simulink model "Timers"  (R2025a)
settings: Solver=FixedStepDiscrete  StartTime=0  StopTime=1  FixedStep=1e-7  RelTol=1e-3
libraries: simulink_extras x216, simulink x13
(part 4 of 7)

== system Timers/Eg: Prescaler/Counter ==
  INC : Inport
  TC_RST : Inport  Port=2
  Constant : Constant
  D Flip-Flop{1..7,11} (8 alike) : simulink_extras/Flip Flops/D Flip-Flop
  Delay One Step : Delay  DelayLength=1
  Demux : Demux  Outputs=8
  Half Adder : Subsystem
      settings: PortSchema="{\"entries\":[{\"content\":{\"sides\":[{\"content\":{\"connectorIds\":[\"In1\"]},\"type\":\"ConnectorPlacement.EquallySpacedRectSide\",\"uuid\":\"d3a7e232-15f2-47a9-a065-9480c81dc57e\"},{\"content\":{\"connectorIds\":[\"Out1\"],\"side\":\"RIGHT\"},\"type\":\"ConnectorPlacement.EquallySpacedRectSide\",\"uuid\":\"e118f150-fee7-4aeb-941e-53c3f02c6791\"},{\"content\":{\"connectorIds\":[\"Out2\"],\"side\":\"TOP\"},\"type\":\"ConnectorPlacement.EquallySpacedRectSide\",\"uuid\":\"6d9038ab-faad-455b-a9c5-8fe0bbf34e51\"},{\"content\":{\"connectorIds\":[\"In2\"],\"side\":\"BOTTOM\"},\"type\":\"ConnectorPlacement.EquallySpacedRectSide\",\"uuid\":\"d09c8d4f-08f3-4c52-88a6-8c6db517fc7a\"}]},\"type\":\"ConnectorPlacement.EquallySpacedConnector\",\"uuid\":\"5bc947ce-f1cd-4957-9186-40c14c78de7d\"}],\"packageUris\":[\"http://schema.mathworks.com/mf0/Connector/R2020b\"],\"version\":\"1.0\"}"
  Half Adder1 : Subsystem
      settings: PortSchema="{\"entries\":[{\"content\":{\"sides\":[{\"content\":{\"connectorIds\":[\"In1\"]},\"type\":\"ConnectorPlacement.EquallySpacedRectSide\",\"uuid\":\"d3a7e232-15f2-47a9-a065-9480c81dc57e\"},{\"content\":{\"connectorIds\":[\"Out1\"],\"side\":\"RIGHT\"},\"type\":\"ConnectorPlacement.EquallySpacedRectSide\",\"uuid\":\"e118f150-fee7-4aeb-941e-53c3f02c6791\"},{\"content\":{\"connectorIds\":[\"Out2\"],\"side\":\"TOP\"},\"type\":\"ConnectorPlacement.EquallySpacedRectSide\",\"uuid\":\"6d9038ab-faad-455b-a9c5-8fe0bbf34e51\"},{\"content\":{\"connectorIds\":[\"In2\"],\"side\":\"BOTTOM\"},\"type\":\"ConnectorPlacement.EquallySpacedRectSide\",\"uuid\":\"d09c8d4f-08f3-4c52-88a6-8c6db517fc7a\"}]},\"type\":\"ConnectorPlacement.EquallySpacedConnector\",\"uuid\":\"5bc947ce-f1cd-4957-9186-40c14c78de7d\"}],\"packageUris\":[\"http://schema.mathworks.com/mf0/Connector/R2020b\"],\"version\":\"1.0\"}"
  Half Adder2 : Subsystem
      settings: PortSchema="{\"entries\":[{\"content\":{\"sides\":[{\"content\":{\"connectorIds\":[\"In1\"]},\"type\":\"ConnectorPlacement.EquallySpacedRectSide\",\"uuid\":\"d3a7e232-15f2-47a9-a065-9480c81dc57e\"},{\"content\":{\"connectorIds\":[\"Out1\"],\"side\":\"RIGHT\"},\"type\":\"ConnectorPlacement.EquallySpacedRectSide\",\"uuid\":\"e118f150-fee7-4aeb-941e-53c3f02c6791\"},{\"content\":{\"connectorIds\":[\"Out2\"],\"side\":\"TOP\"},\"type\":\"ConnectorPlacement.EquallySpacedRectSide\",\"uuid\":\"6d9038ab-faad-455b-a9c5-8fe0bbf34e51\"},{\"content\":{\"connectorIds\":[\"In2\"],\"side\":\"BOTTOM\"},\"type\":\"ConnectorPlacement.EquallySpacedRectSide\",\"uuid\":\"d09c8d4f-08f3-4c52-88a6-8c6db517fc7a\"}]},\"type\":\"ConnectorPlacement.EquallySpacedConnector\",\"uuid\":\"5bc947ce-f1cd-4957-9186-40c14c78de7d\"}],\"packageUris\":[\"http://schema.mathworks.com/mf0/Connector/R2020b\"],\"version\":\"1.0\"}"
  Half Adder3 : Subsystem
      settings: PortSchema="{\"entries\":[{\"content\":{\"sides\":[{\"content\":{\"connectorIds\":[\"In1\"]},\"type\":\"ConnectorPlacement.EquallySpacedRectSide\",\"uuid\":\"d3a7e232-15f2-47a9-a065-9480c81dc57e\"},{\"content\":{\"connectorIds\":[\"Out1\"],\"side\":\"RIGHT\"},\"type\":\"ConnectorPlacement.EquallySpacedRectSide\",\"uuid\":\"e118f150-fee7-4aeb-941e-53c3f02c6791\"},{\"content\":{\"connectorIds\":[\"Out2\"],\"side\":\"TOP\"},\"type\":\"ConnectorPlacement.EquallySpacedRectSide\",\"uuid\":\"6d9038ab-faad-455b-a9c5-8fe0bbf34e51\"},{\"content\":{\"connectorIds\":[\"In2\"],\"side\":\"BOTTOM\"},\"type\":\"ConnectorPlacement.EquallySpacedRectSide\",\"uuid\":\"d09c8d4f-08f3-4c52-88a6-8c6db517fc7a\"}]},\"type\":\"ConnectorPlacement.EquallySpacedConnector\",\"uuid\":\"5bc947ce-f1cd-4957-9186-40c14c78de7d\"}],\"packageUris\":[\"http://schema.mathworks.com/mf0/Connector/R2020b\"],\"version\":\"1.0\"}"
  Half Adder4 : Subsystem
      settings: PortSchema="{\"entries\":[{\"content\":{\"sides\":[{\"content\":{\"connectorIds\":[\"In1\"]},\"type\":\"ConnectorPlacement.EquallySpacedRectSide\",\"uuid\":\"d3a7e232-15f2-47a9-a065-9480c81dc57e\"},{\"content\":{\"connectorIds\":[\"Out1\"],\"side\":\"RIGHT\"},\"type\":\"ConnectorPlacement.EquallySpacedRectSide\",\"uuid\":\"e118f150-fee7-4aeb-941e-53c3f02c6791\"},{\"content\":{\"connectorIds\":[\"Out2\"],\"side\":\"TOP\"},\"type\":\"ConnectorPlacement.EquallySpacedRectSide\",\"uuid\":\"6d9038ab-faad-455b-a9c5-8fe0bbf34e51\"},{\"content\":{\"connectorIds\":[\"In2\"],\"side\":\"BOTTOM\"},\"type\":\"ConnectorPlacement.EquallySpacedRectSide\",\"uuid\":\"d09c8d4f-08f3-4c52-88a6-8c6db517fc7a\"}]},\"type\":\"ConnectorPlacement.EquallySpacedConnector\",\"uuid\":\"5bc947ce-f1cd-4957-9186-40c14c78de7d\"}],\"packageUris\":[\"http://schema.mathworks.com/mf0/Connector/R2020b\"],\"version\":\"1.0\"}"
  Half Adder5 : Subsystem
      settings: PortSchema="{\"entries\":[{\"content\":{\"sides\":[{\"content\":{\"connectorIds\":[\"In1\"]},\"type\":\"ConnectorPlacement.EquallySpacedRectSide\",\"uuid\":\"d3a7e232-15f2-47a9-a065-9480c81dc57e\"},{\"content\":{\"connectorIds\":[\"Out1\"],\"side\":\"RIGHT\"},\"type\":\"ConnectorPlacement.EquallySpacedRectSide\",\"uuid\":\"e118f150-fee7-4aeb-941e-53c3f02c6791\"},{\"content\":{\"connectorIds\":[\"Out2\"],\"side\":\"TOP\"},\"type\":\"ConnectorPlacement.EquallySpacedRectSide\",\"uuid\":\"6d9038ab-faad-455b-a9c5-8fe0bbf34e51\"},{\"content\":{\"connectorIds\":[\"In2\"],\"side\":\"BOTTOM\"},\"type\":\"ConnectorPlacement.EquallySpacedRectSide\",\"uuid\":\"d09c8d4f-08f3-4c52-88a6-8c6db517fc7a\"}]},\"type\":\"ConnectorPlacement.EquallySpacedConnector\",\"uuid\":\"5bc947ce-f1cd-4957-9186-40c14c78de7d\"}],\"packageUris\":[\"http://schema.mathworks.com/mf0/Connector/R2020b\"],\"version\":\"1.0\"}"
  Half Adder6 : Subsystem
      settings: PortSchema="{\"entries\":[{\"content\":{\"sides\":[{\"content\":{\"connectorIds\":[\"In1\"]},\"type\":\"ConnectorPlacement.EquallySpacedRectSide\",\"uuid\":\"d3a7e232-15f2-47a9-a065-9480c81dc57e\"},{\"content\":{\"connectorIds\":[\"Out1\"],\"side\":\"RIGHT\"},\"type\":\"ConnectorPlacement.EquallySpacedRectSide\",\"uuid\":\"e118f150-fee7-4aeb-941e-53c3f02c6791\"},{\"content\":{\"side\":\"TOP\"},\"type\":\"ConnectorPlacement.EquallySpacedRectSide\",\"uuid\":\"6d9038ab-faad-455b-a9c5-8fe0bbf34e51\"},{\"content\":{\"connectorIds\":[\"In2\"],\"side\":\"BOTTOM\"},\"type\":\"ConnectorPlacement.EquallySpacedRectSide\",\"uuid\":\"d09c8d4f-08f3-4c52-88a6-8c6db517fc7a\"}]},\"type\":\"ConnectorPlacement.EquallySpacedConnector\",\"uuid\":\"5bc947ce-f1cd-4957-9186-40c14c78de7d\"}],\"packageUris\":[\"http://schema.mathworks.com/mf0/Connector/R2020b\"],\"version\":\"1.0\"}"
  Half Adder7 : Subsystem
      settings: PortSchema="{\"entries\":[{\"content\":{\"sides\":[{\"content\":{\"connectorIds\":[\"In1\"]},\"type\":\"ConnectorPlacement.EquallySpacedRectSide\",\"uuid\":\"d3a7e232-15f2-47a9-a065-9480c81dc57e\"},{\"content\":{\"connectorIds\":[\"Out1\"],\"side\":\"RIGHT\"},\"type\":\"ConnectorPlacement.EquallySpacedRectSide\",\"uuid\":\"e118f150-fee7-4aeb-941e-53c3f02c6791\"},{\"content\":{\"connectorIds\":[\"Out2\"],\"side\":\"TOP\"},\"type\":\"ConnectorPlacement.EquallySpacedRectSide\",\"uuid\":\"6d9038ab-faad-455b-a9c5-8fe0bbf34e51\"},{\"content\":{\"connectorIds\":[\"In2\"],\"side\":\"BOTTOM\"},\"type\":\"ConnectorPlacement.EquallySpacedRectSide\",\"uuid\":\"d09c8d4f-08f3-4c52-88a6-8c6db517fc7a\"}]},\"type\":\"ConnectorPlacement.EquallySpacedConnector\",\"uuid\":\"5bc947ce-f1cd-4957-9186-40c14c78de7d\"}],\"packageUris\":[\"http://schema.mathworks.com/mf0/Connector/R2020b\"],\"version\":\"1.0\"}"
  Mux1 : Mux  Inputs=8
  Mux2 : Mux  Inputs=8
  NOT : Logic  Operator=NOT  IconShape=distinctive  AllPortsSameDT=off  OutDataTypeStr=boolean
  TC : Outport
  wires:
  Mux1/1 -> Delay One Step/1
  TC_RST/1 -> NOT/1
  Delay One Step/1 -> Demux/1
  Demux/4 -> D Flip-Flop4/1
  Demux/3 -> D Flip-Flop2/1
  Demux/2 -> D Flip-Flop3/1
  Demux/1 -> D Flip-Flop1/1
  Demux/8 -> D Flip-Flop7/1
  Demux/7 -> D Flip-Flop5/1
  Demux/6 -> D Flip-Flop6/1
  Demux/5 -> D Flip-Flop11/1
  INC/1 -> D Flip-Flop2/2, D Flip-Flop3/2, D Flip-Flop1/2, D Flip-Flop4/2, D Flip-Flop11/2, D Flip-Flop6/2, D Flip-Flop5/2, D Flip-Flop7/2
  Constant/1 -> Half Adder7/2("B ")
  Half Adder5/2(Carry) -> Half Adder6/2("B ")
  Half Adder/2(Carry) -> Half Adder1/2("B ")
  Half Adder4/1(Sum) -> Mux1/3
  Half Adder6/1(Sum) -> Mux1/1
  Half Adder5/1(Sum) -> Mux1/2
  Half Adder1/1(Sum) -> Mux1/6
  Half Adder/1(Sum) -> Mux1/7
  Half Adder2/1(Sum) -> Mux1/5
  Half Adder2/2(Carry) -> Half Adder3/2("B ")
  Half Adder3/1(Sum) -> Mux1/4
  Half Adder4/2(Carry) -> Half Adder5/2("B ")
  Half Adder3/2(Carry) -> Half Adder4/2("B ")
  Half Adder1/2(Carry) -> Half Adder2/2("B ")
  Half Adder7/1(Sum) -> Mux1/8
  Half Adder7/2(Carry) -> Half Adder/2("B ")
  D Flip-Flop1/1 -> Mux2/1, Half Adder6/1(A)  "D1"
  D Flip-Flop3/1 -> Mux2/2, Half Adder5/1(A)  "D3"
  D Flip-Flop2/1 -> Mux2/3, Half Adder4/1(A)  "D4"
  D Flip-Flop4/1 -> Mux2/4, Half Adder3/1(A)  "D2"
  D Flip-Flop11/1 -> Mux2/5, Half Adder2/1(A)  "D1"
  D Flip-Flop6/1 -> Mux2/6, Half Adder1/1(A)  "D3"
  D Flip-Flop5/1 -> Mux2/7, Half Adder/1(A)  "D4"
  D Flip-Flop7/1 -> Mux2/8, Half Adder7/1(A)  "D2"
  Mux2/1 -> TC/1
  NOT/1 -> D Flip-Flop2/3, D Flip-Flop1/3, D Flip-Flop3/3, D Flip-Flop4/3, D Flip-Flop11/3, D Flip-Flop6/3, D Flip-Flop5/3, D Flip-Flop7/3

== system Timers/Eg: Prescaler/Counter1 ==
  INC : Inport
  TC_RST : Inport  Port=2
  Constant : Constant
  D Flip-Flop{1..7,11} (8 alike) : simulink_extras/Flip Flops/D Flip-Flop
  Demux : Demux  Outputs=8
  Half Adder : Subsystem
      settings: PortSchema="{\"entries\":[{\"content\":{\"sides\":[{\"content\":{\"connectorIds\":[\"In1\"]},\"type\":\"ConnectorPlacement.EquallySpacedRectSide\",\"uuid\":\"d3a7e232-15f2-47a9-a065-9480c81dc57e\"},{\"content\":{\"connectorIds\":[\"Out1\"],\"side\":\"RIGHT\"},\"type\":\"ConnectorPlacement.EquallySpacedRectSide\",\"uuid\":\"e118f150-fee7-4aeb-941e-53c3f02c6791\"},{\"content\":{\"connectorIds\":[\"Out2\"],\"side\":\"TOP\"},\"type\":\"ConnectorPlacement.EquallySpacedRectSide\",\"uuid\":\"6d9038ab-faad-455b-a9c5-8fe0bbf34e51\"},{\"content\":{\"connectorIds\":[\"In2\"],\"side\":\"BOTTOM\"},\"type\":\"ConnectorPlacement.EquallySpacedRectSide\",\"uuid\":\"d09c8d4f-08f3-4c52-88a6-8c6db517fc7a\"}]},\"type\":\"ConnectorPlacement.EquallySpacedConnector\",\"uuid\":\"5bc947ce-f1cd-4957-9186-40c14c78de7d\"}],\"packageUris\":[\"http://schema.mathworks.com/mf0/Connector/R2020b\"],\"version\":\"1.0\"}"
  Half Adder1 : Subsystem
      settings: PortSchema="{\"entries\":[{\"content\":{\"sides\":[{\"content\":{\"connectorIds\":[\"In1\"]},\"type\":\"ConnectorPlacement.EquallySpacedRectSide\",\"uuid\":\"d3a7e232-15f2-47a9-a065-9480c81dc57e\"},{\"content\":{\"connectorIds\":[\"Out1\"],\"side\":\"RIGHT\"},\"type\":\"ConnectorPlacement.EquallySpacedRectSide\",\"uuid\":\"e118f150-fee7-4aeb-941e-53c3f02c6791\"},{\"content\":{\"connectorIds\":[\"Out2\"],\"side\":\"TOP\"},\"type\":\"ConnectorPlacement.EquallySpacedRectSide\",\"uuid\":\"6d9038ab-faad-455b-a9c5-8fe0bbf34e51\"},{\"content\":{\"connectorIds\":[\"In2\"],\"side\":\"BOTTOM\"},\"type\":\"ConnectorPlacement.EquallySpacedRectSide\",\"uuid\":\"d09c8d4f-08f3-4c52-88a6-8c6db517fc7a\"}]},\"type\":\"ConnectorPlacement.EquallySpacedConnector\",\"uuid\":\"5bc947ce-f1cd-4957-9186-40c14c78de7d\"}],\"packageUris\":[\"http://schema.mathworks.com/mf0/Connector/R2020b\"],\"version\":\"1.0\"}"
  Half Adder2 : Subsystem
      settings: PortSchema="{\"entries\":[{\"content\":{\"sides\":[{\"content\":{\"connectorIds\":[\"In1\"]},\"type\":\"ConnectorPlacement.EquallySpacedRectSide\",\"uuid\":\"d3a7e232-15f2-47a9-a065-9480c81dc57e\"},{\"content\":{\"connectorIds\":[\"Out1\"],\"side\":\"RIGHT\"},\"type\":\"ConnectorPlacement.EquallySpacedRectSide\",\"uuid\":\"e118f150-fee7-4aeb-941e-53c3f02c6791\"},{\"content\":{\"connectorIds\":[\"Out2\"],\"side\":\"TOP\"},\"type\":\"ConnectorPlacement.EquallySpacedRectSide\",\"uuid\":\"6d9038ab-faad-455b-a9c5-8fe0bbf34e51\"},{\"content\":{\"connectorIds\":[\"In2\"],\"side\":\"BOTTOM\"},\"type\":\"ConnectorPlacement.EquallySpacedRectSide\",\"uuid\":\"d09c8d4f-08f3-4c52-88a6-8c6db517fc7a\"}]},\"type\":\"ConnectorPlacement.EquallySpacedConnector\",\"uuid\":\"5bc947ce-f1cd-4957-9186-40c14c78de7d\"}],\"packageUris\":[\"http://schema.mathworks.com/mf0/Connector/R2020b\"],\"version\":\"1.0\"}"
  Half Adder3 : Subsystem
      settings: PortSchema="{\"entries\":[{\"content\":{\"sides\":[{\"content\":{\"connectorIds\":[\"In1\"]},\"type\":\"ConnectorPlacement.EquallySpacedRectSide\",\"uuid\":\"d3a7e232-15f2-47a9-a065-9480c81dc57e\"},{\"content\":{\"connectorIds\":[\"Out1\"],\"side\":\"RIGHT\"},\"type\":\"ConnectorPlacement.EquallySpacedRectSide\",\"uuid\":\"e118f150-fee7-4aeb-941e-53c3f02c6791\"},{\"content\":{\"connectorIds\":[\"Out2\"],\"side\":\"TOP\"},\"type\":\"ConnectorPlacement.EquallySpacedRectSide\",\"uuid\":\"6d9038ab-faad-455b-a9c5-8fe0bbf34e51\"},{\"content\":{\"connectorIds\":[\"In2\"],\"side\":\"BOTTOM\"},\"type\":\"ConnectorPlacement.EquallySpacedRectSide\",\"uuid\":\"d09c8d4f-08f3-4c52-88a6-8c6db517fc7a\"}]},\"type\":\"ConnectorPlacement.EquallySpacedConnector\",\"uuid\":\"5bc947ce-f1cd-4957-9186-40c14c78de7d\"}],\"packageUris\":[\"http://schema.mathworks.com/mf0/Connector/R2020b\"],\"version\":\"1.0\"}"
  Half Adder4 : Subsystem
      settings: PortSchema="{\"entries\":[{\"content\":{\"sides\":[{\"content\":{\"connectorIds\":[\"In1\"]},\"type\":\"ConnectorPlacement.EquallySpacedRectSide\",\"uuid\":\"d3a7e232-15f2-47a9-a065-9480c81dc57e\"},{\"content\":{\"connectorIds\":[\"Out1\"],\"side\":\"RIGHT\"},\"type\":\"ConnectorPlacement.EquallySpacedRectSide\",\"uuid\":\"e118f150-fee7-4aeb-941e-53c3f02c6791\"},{\"content\":{\"connectorIds\":[\"Out2\"],\"side\":\"TOP\"},\"type\":\"ConnectorPlacement.EquallySpacedRectSide\",\"uuid\":\"6d9038ab-faad-455b-a9c5-8fe0bbf34e51\"},{\"content\":{\"connectorIds\":[\"In2\"],\"side\":\"BOTTOM\"},\"type\":\"ConnectorPlacement.EquallySpacedRectSide\",\"uuid\":\"d09c8d4f-08f3-4c52-88a6-8c6db517fc7a\"}]},\"type\":\"ConnectorPlacement.EquallySpacedConnector\",\"uuid\":\"5bc947ce-f1cd-4957-9186-40c14c78de7d\"}],\"packageUris\":[\"http://schema.mathworks.com/mf0/Connector/R2020b\"],\"version\":\"1.0\"}"
  Half Adder5 : Subsystem
      settings: PortSchema="{\"entries\":[{\"content\":{\"sides\":[{\"content\":{\"connectorIds\":[\"In1\"]},\"type\":\"ConnectorPlacement.EquallySpacedRectSide\",\"uuid\":\"d3a7e232-15f2-47a9-a065-9480c81dc57e\"},{\"content\":{\"connectorIds\":[\"Out1\"],\"side\":\"RIGHT\"},\"type\":\"ConnectorPlacement.EquallySpacedRectSide\",\"uuid\":\"e118f150-fee7-4aeb-941e-53c3f02c6791\"},{\"content\":{\"connectorIds\":[\"Out2\"],\"side\":\"TOP\"},\"type\":\"ConnectorPlacement.EquallySpacedRectSide\",\"uuid\":\"6d9038ab-faad-455b-a9c5-8fe0bbf34e51\"},{\"content\":{\"connectorIds\":[\"In2\"],\"side\":\"BOTTOM\"},\"type\":\"ConnectorPlacement.EquallySpacedRectSide\",\"uuid\":\"d09c8d4f-08f3-4c52-88a6-8c6db517fc7a\"}]},\"type\":\"ConnectorPlacement.EquallySpacedConnector\",\"uuid\":\"5bc947ce-f1cd-4957-9186-40c14c78de7d\"}],\"packageUris\":[\"http://schema.mathworks.com/mf0/Connector/R2020b\"],\"version\":\"1.0\"}"
  Half Adder6 : Subsystem
      settings: PortSchema="{\"entries\":[{\"content\":{\"sides\":[{\"content\":{\"connectorIds\":[\"In1\"]},\"type\":\"ConnectorPlacement.EquallySpacedRectSide\",\"uuid\":\"d3a7e232-15f2-47a9-a065-9480c81dc57e\"},{\"content\":{\"connectorIds\":[\"Out1\"],\"side\":\"RIGHT\"},\"type\":\"ConnectorPlacement.EquallySpacedRectSide\",\"uuid\":\"e118f150-fee7-4aeb-941e-53c3f02c6791\"},{\"content\":{\"side\":\"TOP\"},\"type\":\"ConnectorPlacement.EquallySpacedRectSide\",\"uuid\":\"6d9038ab-faad-455b-a9c5-8fe0bbf34e51\"},{\"content\":{\"connectorIds\":[\"In2\"],\"side\":\"BOTTOM\"},\"type\":\"ConnectorPlacement.EquallySpacedRectSide\",\"uuid\":\"d09c8d4f-08f3-4c52-88a6-8c6db517fc7a\"}]},\"type\":\"ConnectorPlacement.EquallySpacedConnector\",\"uuid\":\"5bc947ce-f1cd-4957-9186-40c14c78de7d\"}],\"packageUris\":[\"http://schema.mathworks.com/mf0/Connector/R2020b\"],\"version\":\"1.0\"}"
  Half Adder7 : Subsystem
      settings: PortSchema="{\"entries\":[{\"content\":{\"sides\":[{\"content\":{\"connectorIds\":[\"In1\"]},\"type\":\"ConnectorPlacement.EquallySpacedRectSide\",\"uuid\":\"d3a7e232-15f2-47a9-a065-9480c81dc57e\"},{\"content\":{\"connectorIds\":[\"Out1\"],\"side\":\"RIGHT\"},\"type\":\"ConnectorPlacement.EquallySpacedRectSide\",\"uuid\":\"e118f150-fee7-4aeb-941e-53c3f02c6791\"},{\"content\":{\"connectorIds\":[\"Out2\"],\"side\":\"TOP\"},\"type\":\"ConnectorPlacement.EquallySpacedRectSide\",\"uuid\":\"6d9038ab-faad-455b-a9c5-8fe0bbf34e51\"},{\"content\":{\"connectorIds\":[\"In2\"],\"side\":\"BOTTOM\"},\"type\":\"ConnectorPlacement.EquallySpacedRectSide\",\"uuid\":\"d09c8d4f-08f3-4c52-88a6-8c6db517fc7a\"}]},\"type\":\"ConnectorPlacement.EquallySpacedConnector\",\"uuid\":\"5bc947ce-f1cd-4957-9186-40c14c78de7d\"}],\"packageUris\":[\"http://schema.mathworks.com/mf0/Connector/R2020b\"],\"version\":\"1.0\"}"
  Mux1 : Mux  Inputs=8
  Mux2 : Mux  Inputs=8
  NOT : Logic  Operator=NOT  IconShape=distinctive  AllPortsSameDT=off  OutDataTypeStr=boolean
  TC : Outport
  wires:
  TC_RST/1 -> NOT/1
  Mux1/1 -> Demux/1
  Demux/4 -> D Flip-Flop4/1
  Demux/3 -> D Flip-Flop2/1
  Demux/2 -> D Flip-Flop3/1
  Demux/1 -> D Flip-Flop1/1
  Demux/8 -> D Flip-Flop7/1
  Demux/7 -> D Flip-Flop5/1
  Demux/6 -> D Flip-Flop6/1
  Demux/5 -> D Flip-Flop11/1
  INC/1 -> D Flip-Flop2/2, D Flip-Flop3/2, D Flip-Flop1/2, D Flip-Flop4/2, D Flip-Flop11/2, D Flip-Flop6/2, D Flip-Flop5/2, D Flip-Flop7/2
  Constant/1 -> Half Adder7/2("B ")
  Half Adder5/2(Carry) -> Half Adder6/2("B ")
  Half Adder/2(Carry) -> Half Adder1/2("B ")
  Half Adder4/1(Sum) -> Mux1/3
  Half Adder6/1(Sum) -> Mux1/1
  Half Adder5/1(Sum) -> Mux1/2
  Half Adder1/1(Sum) -> Mux1/6
  Half Adder/1(Sum) -> Mux1/7
  Half Adder2/1(Sum) -> Mux1/5
  Half Adder2/2(Carry) -> Half Adder3/2("B ")
  Half Adder3/1(Sum) -> Mux1/4
  Half Adder4/2(Carry) -> Half Adder5/2("B ")
  Half Adder3/2(Carry) -> Half Adder4/2("B ")
  Half Adder1/2(Carry) -> Half Adder2/2("B ")
  Half Adder7/1(Sum) -> Mux1/8
  Half Adder7/2(Carry) -> Half Adder/2("B ")
  D Flip-Flop1/1 -> Mux2/1, Half Adder6/1(A)  "D1"
  D Flip-Flop3/1 -> Mux2/2, Half Adder5/1(A)  "D3"
  D Flip-Flop2/1 -> Mux2/3, Half Adder4/1(A)  "D4"
  D Flip-Flop4/1 -> Mux2/4, Half Adder3/1(A)  "D2"
  D Flip-Flop11/1 -> Mux2/5, Half Adder2/1(A)  "D1"
  D Flip-Flop6/1 -> Mux2/6, Half Adder1/1(A)  "D3"
  D Flip-Flop5/1 -> Mux2/7, Half Adder/1(A)  "D4"
  D Flip-Flop7/1 -> Mux2/8, Half Adder7/1(A)  "D2"
  Mux2/1 -> TC/1
  NOT/1 -> D Flip-Flop2/3, D Flip-Flop1/3, D Flip-Flop3/3, D Flip-Flop4/3, D Flip-Flop11/3, D Flip-Flop6/3, D Flip-Flop5/3, D Flip-Flop7/3

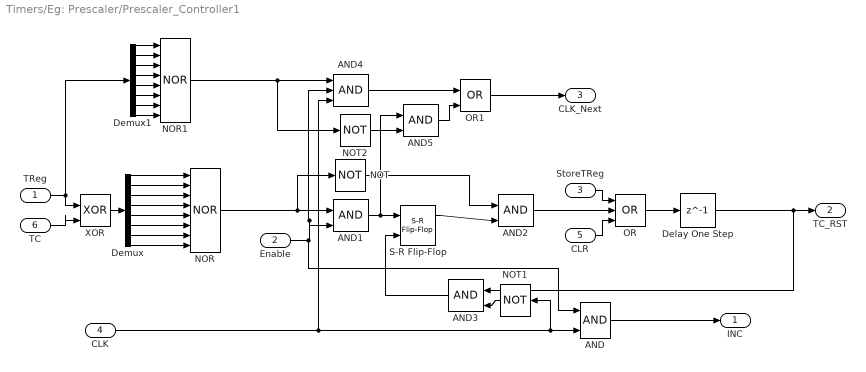
== system Timers/Eg: Prescaler/Prescaler_Controller1 ==
  TReg : Inport
  Enable : Inport  Port=2
  StoreTReg : Inport  Port=3
  CLK : Inport  Port=4
  "CLR " : Inport  Port=5
  TC : Inport  Port=6
  AND{,1..3,5} (5 alike) : Logic  IconShape=distinctive  AllPortsSameDT=off  OutDataTypeStr=boolean
  AND4 : Logic  Inputs=3  IconShape=distinctive  AllPortsSameDT=off  OutDataTypeStr=boolean
  Delay One Step : Delay  DelayLength=1  SampleTime=1e-6
  Demux : Demux  Outputs=8
  Demux1 : Demux  Outputs=8
  NOR : Logic  Operator=NOR  Inputs=8  IconShape=distinctive  AllPortsSameDT=off  OutDataTypeStr=boolean
  NOR1 : Logic  Operator=NOR  Inputs=8  IconShape=distinctive  AllPortsSameDT=off  OutDataTypeStr=boolean
  NOT : Logic  Operator=NOT  IconShape=distinctive  AllPortsSameDT=off  OutDataTypeStr=boolean
  NOT1 : Logic  Operator=NOT  IconShape=distinctive  AllPortsSameDT=off  OutDataTypeStr=boolean
  NOT2 : Logic  Operator=NOT  IconShape=distinctive  AllPortsSameDT=off  OutDataTypeStr=boolean
  OR : Logic  Operator=OR  Inputs=3  IconShape=distinctive  AllPortsSameDT=off  OutDataTypeStr=boolean
  OR1 : Logic  Operator=OR  IconShape=distinctive  AllPortsSameDT=off  OutDataTypeStr=boolean
  S-R Flip-Flop : simulink_extras/Flip Flops/S-R Flip-Flop  initial_condition=0
  XOR : Logic  Operator=XOR  IconShape=distinctive  AllPortsSameDT=off  OutDataTypeStr=boolean
  INC : Outport
  TC_RST : Outport  Port=2
  CLK_Next : Outport  Port=3
  wires:
  Enable/1 -> AND4/2, AND1/2, AND/1
  Delay One Step/1 -> TC_RST/1, AND3/1
  Demux/3 -> NOR/3
  CLK/1 -> AND4/3, NOT1/1, AND/2
  AND/1 -> INC/1
  Demux/6 -> NOR/6
  Demux/1 -> NOR/1
  Demux/8 -> NOR/8
  StoreTReg/1 -> OR/1
  TC/1 -> XOR/2
  "CLR "/1 -> OR/3
  AND3/1 -> S-R Flip-Flop/2
  Demux/4 -> NOR/4
  OR/1 -> Delay One Step/1
  Demux/5 -> NOR/5
  TReg/1 -> XOR/1, Demux1/1
  NOT1/1 -> AND3/2
  Demux/2 -> NOR/2
  AND1/1 -> AND5/1, S-R Flip-Flop/1
  NOT/1 -> AND2/1
  Demux/7 -> NOR/7
  NOR/1 -> NOT/1, AND1/1
  XOR/1 -> Demux/1
  S-R Flip-Flop/1 -> AND2/2
  AND2/1 -> OR/2
  Demux1/8 -> NOR1/8
  Demux1/3 -> NOR1/3
  Demux1/1 -> NOR1/1
  Demux1/2 -> NOR1/2
  Demux1/4 -> NOR1/4
  Demux1/5 -> NOR1/5
  Demux1/6 -> NOR1/6
  Demux1/7 -> NOR1/7
  NOR1/1 -> NOT2/1, AND4/1
  AND4/1 -> OR1/1
  OR1/1 -> CLK_Next/1
  AND5/1 -> OR1/2
  NOT2/1 -> AND5/2

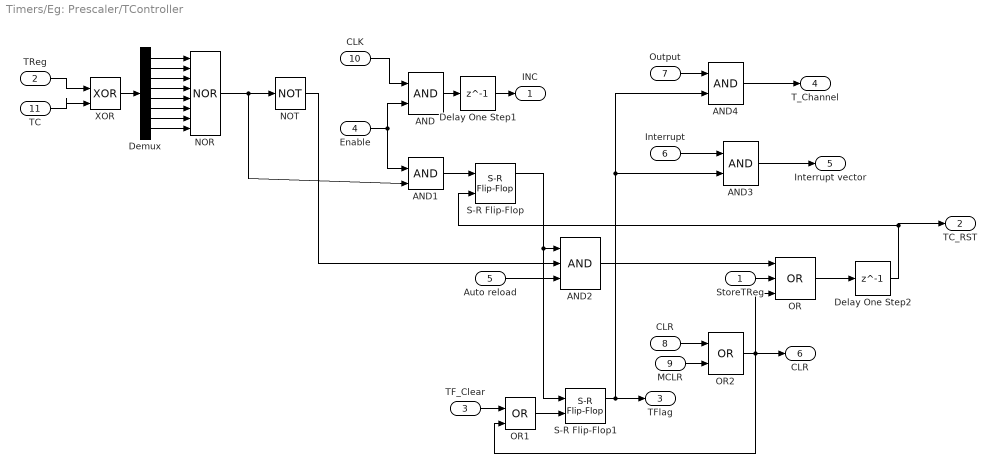
== system Timers/Eg: Prescaler/TController ==
  StoreTReg : Inport
  TReg : Inport  Port=2
  TF_Clear : Inport  Port=3
  Enable : Inport  Port=4
  Auto reload : Inport  Port=5
  Interrupt : Inport  Port=6
  Output : Inport  Port=7
  "CLR " : Inport  Port=8
  MCLR : Inport  Port=9
  CLK : Inport  Port=10
  TC : Inport  Port=11
  AND{,1,3..4} (4 alike) : Logic  IconShape=distinctive  AllPortsSameDT=off  OutDataTypeStr=boolean
  AND2 : Logic  Inputs=3  IconShape=distinctive  AllPortsSameDT=off  OutDataTypeStr=boolean
  Delay One Step1 : Delay  DelayLength=1  SampleTime=1e-5
  Delay One Step2 : Delay  DelayLength=1  SampleTime=1e-5
  Demux : Demux  Outputs=8
  NOR : Logic  Operator=NOR  Inputs=8  IconShape=distinctive  AllPortsSameDT=off  OutDataTypeStr=boolean
  NOT : Logic  Operator=NOT  IconShape=distinctive  AllPortsSameDT=off  OutDataTypeStr=boolean
  OR : Logic  Operator=OR  Inputs=3  IconShape=distinctive  AllPortsSameDT=off  OutDataTypeStr=boolean
  OR1 : Logic  Operator=OR  IconShape=distinctive  AllPortsSameDT=off  OutDataTypeStr=boolean
  OR2 : Logic  Operator=OR  IconShape=distinctive  AllPortsSameDT=off  OutDataTypeStr=boolean
  S-R Flip-Flop : simulink_extras/Flip Flops/S-R Flip-Flop  initial_condition=0
  S-R Flip-Flop1 : simulink_extras/Flip Flops/S-R Flip-Flop  initial_condition=0
  XOR : Logic  Operator=XOR  IconShape=distinctive  AllPortsSameDT=off  OutDataTypeStr=boolean
  INC : Outport
  TC_RST : Outport  Port=2
  TFlag : Outport  Port=3
  T_Channel : Outport  Port=4
  Interrupt vector : Outport  Port=5
  CLR : Outport  Port=6
  wires:
  TReg/1 -> XOR/1
  Demux/3 -> NOR/3
  Demux/4 -> NOR/4
  TC/1 -> XOR/2
  XOR/1 -> Demux/1
  Demux/1 -> NOR/1
  Demux/2 -> NOR/2
  Demux/5 -> NOR/5
  Demux/6 -> NOR/6
  Demux/7 -> NOR/7
  Demux/8 -> NOR/8
  NOR/1 -> AND1/2, NOT/1
  Enable/1 -> AND/2, AND1/1
  "CLR "/1 -> OR2/1
  MCLR/1 -> OR2/2
  OR2/1 -> OR/3, CLR/1, OR1/2
  Output/1 -> AND4/1
  Delay One Step2/1 -> TC_RST/1, S-R Flip-Flop/2
  Interrupt/1 -> AND3/1
  AND4/1 -> T_Channel/1
  AND3/1 -> Interrupt vector/1
  NOT/1 -> AND2/2
  CLK/1 -> AND/1
  AND/1 -> Delay One Step1/1
  AND1/1 -> S-R Flip-Flop/1
  S-R Flip-Flop/1 -> S-R Flip-Flop1/1, AND2/1
  AND2/1 -> OR/1
  OR/1 -> Delay One Step2/1
  StoreTReg/1 -> OR/2
  OR1/1 -> S-R Flip-Flop1/2
  TF_Clear/1 -> OR1/1
  S-R Flip-Flop1/1 -> TFlag/1, AND4/2, AND3/2
  Auto reload/1 -> AND2/3
  Delay One Step1/1 -> INC/1

== system Timers/Eg: Prescaler/TPS ==
  Data bus : Inport
  Store : Inport  Port=2
  CLK : Inport  Port=3
  CLR : Inport  Port=4
  Demux : Demux  Outputs=8
  Mux : Mux  Inputs=8
  Subsystem1 : Subsystem
  Subsystem2 : Subsystem
  Subsystem3 : Subsystem
  Subsystem4 : Subsystem
  Subsystem5 : Subsystem
  Subsystem6 : Subsystem
  Subsystem7 : Subsystem
  Subsystem8 : Subsystem
  "Q Bus " : Outport
  wires:
  Demux/4 -> Subsystem2/1(Data)
  Mux/1 -> "Q Bus "/1
  Demux/2 -> Subsystem1/1(Data)
  Data bus/1 -> Demux/1
  Subsystem6/1(Q) -> Mux/8
  Store/1 -> Subsystem1/2(Store), Subsystem4/2(Store), Subsystem2/2(Store), Subsystem7/2(Store), Subsystem5/2(Store), Subsystem6/2(Store), Subsystem8/2(Store), Subsystem3/2(Store)
  Demux/5 -> Subsystem7/1(Data)
  Demux/7 -> Subsystem8/1(Data)
  Demux/3 -> Subsystem4/1(Data)
  Subsystem7/1(Q) -> Mux/5
  Demux/6 -> Subsystem5/1(Data)
  Subsystem1/1(Q) -> Mux/2
  Demux/1 -> Subsystem3/1(Data)
  Subsystem3/1(Q) -> Mux/1
  Demux/8 -> Subsystem6/1(Data)
  Subsystem8/1(Q) -> Mux/7
  Subsystem2/1(Q) -> Mux/4
  Subsystem4/1(Q) -> Mux/3
  Subsystem5/1(Q) -> Mux/6
  CLK/1 -> Subsystem1/3(Clock), Subsystem4/3(Clock), Subsystem2/3(Clock), Subsystem7/3(Clock), Subsystem5/3(Clock), Subsystem6/3(Clock), Subsystem8/3(Clock), Subsystem3/3(Clock)
  CLR/1 -> Subsystem8/4(Clear), Subsystem5/4(Clear), Subsystem7/4(Clear), Subsystem2/4(Clear), Subsystem4/4(Clear), Subsystem1/4(Clear), Subsystem3/4(Clear), Subsystem6/4(Clear)

== system Timers/Eg: Prescaler/TReg ==
  Data bus : Inport
  Store : Inport  Port=2
  CLK : Inport  Port=3
  CLR : Inport  Port=4
  Demux : Demux  Outputs=8
  Mux : Mux  Inputs=8
  Subsystem1 : Subsystem
  Subsystem2 : Subsystem
  Subsystem3 : Subsystem
  Subsystem4 : Subsystem
  Subsystem5 : Subsystem
  Subsystem6 : Subsystem
  Subsystem7 : Subsystem
  Subsystem8 : Subsystem
  "Q Bus " : Outport
  wires:
  Demux/4 -> Subsystem2/1(Data)
  Mux/1 -> "Q Bus "/1
  Demux/2 -> Subsystem1/1(Data)
  Data bus/1 -> Demux/1
  Subsystem6/1(Q) -> Mux/8
  Store/1 -> Subsystem1/2(Store), Subsystem4/2(Store), Subsystem2/2(Store), Subsystem7/2(Store), Subsystem5/2(Store), Subsystem6/2(Store), Subsystem8/2(Store), Subsystem3/2(Store)
  Demux/5 -> Subsystem7/1(Data)
  Demux/7 -> Subsystem8/1(Data)
  Demux/3 -> Subsystem4/1(Data)
  Subsystem7/1(Q) -> Mux/5
  Demux/6 -> Subsystem5/1(Data)
  Subsystem1/1(Q) -> Mux/2
  Demux/1 -> Subsystem3/1(Data)
  Subsystem3/1(Q) -> Mux/1
  Demux/8 -> Subsystem6/1(Data)
  Subsystem8/1(Q) -> Mux/7
  Subsystem2/1(Q) -> Mux/4
  Subsystem4/1(Q) -> Mux/3
  Subsystem5/1(Q) -> Mux/6
  CLK/1 -> Subsystem1/3(Clock), Subsystem4/3(Clock), Subsystem2/3(Clock), Subsystem7/3(Clock), Subsystem5/3(Clock), Subsystem6/3(Clock), Subsystem8/3(Clock), Subsystem3/3(Clock)
  CLR/1 -> Subsystem8/4(Clear), Subsystem5/4(Clear), Subsystem7/4(Clear), Subsystem2/4(Clear), Subsystem4/4(Clear), Subsystem1/4(Clear), Subsystem3/4(Clear), Subsystem6/4(Clear)

== system Timers/Eg: Prescaler/Tcon ==
  Data bus : Inport
  Store : Inport  Port=2
  CLK : Inport  Port=3
  CLR : Inport  Port=4
  Demux : Demux  Outputs=8
  Subsystem1 : Subsystem
  Subsystem2 : Subsystem
  Subsystem3 : Subsystem
  Subsystem4 : Subsystem
  Subsystem5 : Subsystem
  Subsystem6 : Subsystem
  Subsystem7 : Subsystem
  Subsystem8 : Subsystem
  TE : Outport
  TAR : Outport  Port=2
  TI : Outport  Port=3
  TG : Outport  Port=4
  wires:
  Demux/4 -> Subsystem2/1(Data)
  Demux/2 -> Subsystem1/1(Data)
  Data bus/1 -> Demux/1
  Store/1 -> Subsystem1/2(Store), Subsystem4/2(Store), Subsystem2/2(Store), Subsystem7/2(Store), Subsystem5/2(Store), Subsystem6/2(Store), Subsystem8/2(Store), Subsystem3/2(Store)
  Demux/5 -> Subsystem7/1(Data)
  Demux/7 -> Subsystem8/1(Data)
  Demux/3 -> Subsystem4/1(Data)
  Demux/6 -> Subsystem5/1(Data)
  Subsystem1/1(Q) -> TAR/1  "Auto Reload"
  Demux/1 -> Subsystem3/1(Data)
  Subsystem3/1(Q) -> TE/1  "Enabled"
  Demux/8 -> Subsystem6/1(Data)
  CLK/1 -> Subsystem1/3(Clock), Subsystem4/3(Clock), Subsystem2/3(Clock), Subsystem7/3(Clock), Subsystem5/3(Clock), Subsystem6/3(Clock), Subsystem8/3(Clock), Subsystem3/3(Clock)
  CLR/1 -> Subsystem8/4(Clear), Subsystem5/4(Clear), Subsystem7/4(Clear), Subsystem2/4(Clear), Subsystem4/4(Clear), Subsystem1/4(Clear), Subsystem3/4(Clear), Subsystem6/4(Clear)
  Subsystem2/1(Q) -> TG/1  "Interrupt"
  Subsystem4/1(Q) -> TI/1  "Gate"

== system Timers/Eg: Duel Prescaler/Counter/Half Adder ==
  A : Inport
  "B " : Inport  Port=2
  AND : Logic  IconShape=distinctive  AllPortsSameDT=off  OutDataTypeStr=boolean
  XOR : Logic  Operator=XOR  IconShape=distinctive  AllPortsSameDT=off  OutDataTypeStr=boolean
  Sum : Outport
  Carry : Outport  Port=2
  wires:
  A/1 -> AND/1, XOR/1
  "B "/1 -> XOR/2, AND/2
  XOR/1 -> Sum/1
  AND/1 -> Carry/1

== system Timers/Eg: Duel Prescaler/Counter/Half Adder1 ==
  A : Inport
  "B " : Inport  Port=2
  AND : Logic  IconShape=distinctive  AllPortsSameDT=off  OutDataTypeStr=boolean
  XOR : Logic  Operator=XOR  IconShape=distinctive  AllPortsSameDT=off  OutDataTypeStr=boolean
  Sum : Outport
  Carry : Outport  Port=2
  wires:
  A/1 -> AND/1, XOR/1
  "B "/1 -> XOR/2, AND/2
  XOR/1 -> Sum/1
  AND/1 -> Carry/1

== system Timers/Eg: Duel Prescaler/Counter/Half Adder2 ==
  A : Inport
  "B " : Inport  Port=2
  AND : Logic  IconShape=distinctive  AllPortsSameDT=off  OutDataTypeStr=boolean
  XOR : Logic  Operator=XOR  IconShape=distinctive  AllPortsSameDT=off  OutDataTypeStr=boolean
  Sum : Outport
  Carry : Outport  Port=2
  wires:
  A/1 -> AND/1, XOR/1
  "B "/1 -> XOR/2, AND/2
  XOR/1 -> Sum/1
  AND/1 -> Carry/1

== system Timers/Eg: Duel Prescaler/Counter/Half Adder3 ==
  A : Inport
  "B " : Inport  Port=2
  AND : Logic  IconShape=distinctive  AllPortsSameDT=off  OutDataTypeStr=boolean
  XOR : Logic  Operator=XOR  IconShape=distinctive  AllPortsSameDT=off  OutDataTypeStr=boolean
  Sum : Outport
  Carry : Outport  Port=2
  wires:
  A/1 -> AND/1, XOR/1
  "B "/1 -> XOR/2, AND/2
  XOR/1 -> Sum/1
  AND/1 -> Carry/1

== system Timers/Eg: Duel Prescaler/Counter/Half Adder4 ==
  A : Inport
  "B " : Inport  Port=2
  AND : Logic  IconShape=distinctive  AllPortsSameDT=off  OutDataTypeStr=boolean
  XOR : Logic  Operator=XOR  IconShape=distinctive  AllPortsSameDT=off  OutDataTypeStr=boolean
  Sum : Outport
  Carry : Outport  Port=2
  wires:
  A/1 -> AND/1, XOR/1
  "B "/1 -> XOR/2, AND/2
  XOR/1 -> Sum/1
  AND/1 -> Carry/1

== system Timers/Eg: Duel Prescaler/Counter/Half Adder5 ==
  A : Inport
  "B " : Inport  Port=2
  AND : Logic  IconShape=distinctive  AllPortsSameDT=off  OutDataTypeStr=boolean
  XOR : Logic  Operator=XOR  IconShape=distinctive  AllPortsSameDT=off  OutDataTypeStr=boolean
  Sum : Outport
  Carry : Outport  Port=2
  wires:
  A/1 -> AND/1, XOR/1
  "B "/1 -> XOR/2, AND/2
  XOR/1 -> Sum/1
  AND/1 -> Carry/1

== system Timers/Eg: Duel Prescaler/Counter/Half Adder6 ==
  A : Inport
  "B " : Inport  Port=2
  XOR : Logic  Operator=XOR  IconShape=distinctive  AllPortsSameDT=off  OutDataTypeStr=boolean
  Sum : Outport
  wires:
  A/1 -> XOR/1
  "B "/1 -> XOR/2
  XOR/1 -> Sum/1

== system Timers/Eg: Duel Prescaler/Counter/Half Adder7 ==
  A : Inport
  "B " : Inport  Port=2
  AND : Logic  IconShape=distinctive  AllPortsSameDT=off  OutDataTypeStr=boolean
  XOR : Logic  Operator=XOR  IconShape=distinctive  AllPortsSameDT=off  OutDataTypeStr=boolean
  Sum : Outport
  Carry : Outport  Port=2
  wires:
  A/1 -> AND/1, XOR/1
  "B "/1 -> XOR/2, AND/2
  XOR/1 -> Sum/1
  AND/1 -> Carry/1

== system Timers/Eg: Duel Prescaler/Counter1/Half Adder ==
  A : Inport
  "B " : Inport  Port=2
  AND : Logic  IconShape=distinctive  AllPortsSameDT=off  OutDataTypeStr=boolean
  XOR : Logic  Operator=XOR  IconShape=distinctive  AllPortsSameDT=off  OutDataTypeStr=boolean
  Sum : Outport
  Carry : Outport  Port=2
  wires:
  A/1 -> AND/1, XOR/1
  "B "/1 -> XOR/2, AND/2
  XOR/1 -> Sum/1
  AND/1 -> Carry/1

== system Timers/Eg: Duel Prescaler/Counter1/Half Adder1 ==
  A : Inport
  "B " : Inport  Port=2
  AND : Logic  IconShape=distinctive  AllPortsSameDT=off  OutDataTypeStr=boolean
  XOR : Logic  Operator=XOR  IconShape=distinctive  AllPortsSameDT=off  OutDataTypeStr=boolean
  Sum : Outport
  Carry : Outport  Port=2
  wires:
  A/1 -> AND/1, XOR/1
  "B "/1 -> XOR/2, AND/2
  XOR/1 -> Sum/1
  AND/1 -> Carry/1

== system Timers/Eg: Duel Prescaler/Counter1/Half Adder2 ==
  A : Inport
  "B " : Inport  Port=2
  AND : Logic  IconShape=distinctive  AllPortsSameDT=off  OutDataTypeStr=boolean
  XOR : Logic  Operator=XOR  IconShape=distinctive  AllPortsSameDT=off  OutDataTypeStr=boolean
  Sum : Outport
  Carry : Outport  Port=2
  wires:
  A/1 -> AND/1, XOR/1
  "B "/1 -> XOR/2, AND/2
  XOR/1 -> Sum/1
  AND/1 -> Carry/1

== system Timers/Eg: Duel Prescaler/Counter1/Half Adder3 ==
  A : Inport
  "B " : Inport  Port=2
  AND : Logic  IconShape=distinctive  AllPortsSameDT=off  OutDataTypeStr=boolean
  XOR : Logic  Operator=XOR  IconShape=distinctive  AllPortsSameDT=off  OutDataTypeStr=boolean
  Sum : Outport
  Carry : Outport  Port=2
  wires:
  A/1 -> AND/1, XOR/1
  "B "/1 -> XOR/2, AND/2
  XOR/1 -> Sum/1
  AND/1 -> Carry/1

== system Timers/Eg: Duel Prescaler/Counter1/Half Adder4 ==
  A : Inport
  "B " : Inport  Port=2
  AND : Logic  IconShape=distinctive  AllPortsSameDT=off  OutDataTypeStr=boolean
  XOR : Logic  Operator=XOR  IconShape=distinctive  AllPortsSameDT=off  OutDataTypeStr=boolean
  Sum : Outport
  Carry : Outport  Port=2
  wires:
  A/1 -> AND/1, XOR/1
  "B "/1 -> XOR/2, AND/2
  XOR/1 -> Sum/1
  AND/1 -> Carry/1

== system Timers/Eg: Duel Prescaler/Counter1/Half Adder5 ==
  A : Inport
  "B " : Inport  Port=2
  AND : Logic  IconShape=distinctive  AllPortsSameDT=off  OutDataTypeStr=boolean
  XOR : Logic  Operator=XOR  IconShape=distinctive  AllPortsSameDT=off  OutDataTypeStr=boolean
  Sum : Outport
  Carry : Outport  Port=2
  wires:
  A/1 -> AND/1, XOR/1
  "B "/1 -> XOR/2, AND/2
  XOR/1 -> Sum/1
  AND/1 -> Carry/1

== system Timers/Eg: Duel Prescaler/Counter1/Half Adder6 ==
  A : Inport
  "B " : Inport  Port=2
  XOR : Logic  Operator=XOR  IconShape=distinctive  AllPortsSameDT=off  OutDataTypeStr=boolean
  Sum : Outport
  wires:
  A/1 -> XOR/1
  "B "/1 -> XOR/2
  XOR/1 -> Sum/1

== system Timers/Eg: Duel Prescaler/Counter1/Half Adder7 ==
  A : Inport
  "B " : Inport  Port=2
  AND : Logic  IconShape=distinctive  AllPortsSameDT=off  OutDataTypeStr=boolean
  XOR : Logic  Operator=XOR  IconShape=distinctive  AllPortsSameDT=off  OutDataTypeStr=boolean
  Sum : Outport
  Carry : Outport  Port=2
  wires:
  A/1 -> AND/1, XOR/1
  "B "/1 -> XOR/2, AND/2
  XOR/1 -> Sum/1
  AND/1 -> Carry/1

== system Timers/Eg: Duel Prescaler/Counter2/Half Adder ==
  A : Inport
  "B " : Inport  Port=2
  AND : Logic  IconShape=distinctive  AllPortsSameDT=off  OutDataTypeStr=boolean
  XOR : Logic  Operator=XOR  IconShape=distinctive  AllPortsSameDT=off  OutDataTypeStr=boolean
  Sum : Outport
  Carry : Outport  Port=2
  wires:
  A/1 -> AND/1, XOR/1
  "B "/1 -> XOR/2, AND/2
  XOR/1 -> Sum/1
  AND/1 -> Carry/1

== system Timers/Eg: Duel Prescaler/Counter2/Half Adder1 ==
  A : Inport
  "B " : Inport  Port=2
  AND : Logic  IconShape=distinctive  AllPortsSameDT=off  OutDataTypeStr=boolean
  XOR : Logic  Operator=XOR  IconShape=distinctive  AllPortsSameDT=off  OutDataTypeStr=boolean
  Sum : Outport
  Carry : Outport  Port=2
  wires:
  A/1 -> AND/1, XOR/1
  "B "/1 -> XOR/2, AND/2
  XOR/1 -> Sum/1
  AND/1 -> Carry/1

== system Timers/Eg: Duel Prescaler/Counter2/Half Adder2 ==
  A : Inport
  "B " : Inport  Port=2
  AND : Logic  IconShape=distinctive  AllPortsSameDT=off  OutDataTypeStr=boolean
  XOR : Logic  Operator=XOR  IconShape=distinctive  AllPortsSameDT=off  OutDataTypeStr=boolean
  Sum : Outport
  Carry : Outport  Port=2
  wires:
  A/1 -> AND/1, XOR/1
  "B "/1 -> XOR/2, AND/2
  XOR/1 -> Sum/1
  AND/1 -> Carry/1

== system Timers/Eg: Duel Prescaler/Counter2/Half Adder3 ==
  A : Inport
  "B " : Inport  Port=2
  AND : Logic  IconShape=distinctive  AllPortsSameDT=off  OutDataTypeStr=boolean
  XOR : Logic  Operator=XOR  IconShape=distinctive  AllPortsSameDT=off  OutDataTypeStr=boolean
  Sum : Outport
  Carry : Outport  Port=2
  wires:
  A/1 -> AND/1, XOR/1
  "B "/1 -> XOR/2, AND/2
  XOR/1 -> Sum/1
  AND/1 -> Carry/1

== system Timers/Eg: Duel Prescaler/Counter2/Half Adder4 ==
  A : Inport
  "B " : Inport  Port=2
  AND : Logic  IconShape=distinctive  AllPortsSameDT=off  OutDataTypeStr=boolean
  XOR : Logic  Operator=XOR  IconShape=distinctive  AllPortsSameDT=off  OutDataTypeStr=boolean
  Sum : Outport
  Carry : Outport  Port=2
  wires:
  A/1 -> AND/1, XOR/1
  "B "/1 -> XOR/2, AND/2
  XOR/1 -> Sum/1
  AND/1 -> Carry/1

== system Timers/Eg: Duel Prescaler/Counter2/Half Adder5 ==
  A : Inport
  "B " : Inport  Port=2
  AND : Logic  IconShape=distinctive  AllPortsSameDT=off  OutDataTypeStr=boolean
  XOR : Logic  Operator=XOR  IconShape=distinctive  AllPortsSameDT=off  OutDataTypeStr=boolean
  Sum : Outport
  Carry : Outport  Port=2
  wires:
  A/1 -> AND/1, XOR/1
  "B "/1 -> XOR/2, AND/2
  XOR/1 -> Sum/1
  AND/1 -> Carry/1

== system Timers/Eg: Duel Prescaler/Counter2/Half Adder6 ==
  A : Inport
  "B " : Inport  Port=2
  XOR : Logic  Operator=XOR  IconShape=distinctive  AllPortsSameDT=off  OutDataTypeStr=boolean
  Sum : Outport
  wires:
  A/1 -> XOR/1
  "B "/1 -> XOR/2
  XOR/1 -> Sum/1

== system Timers/Eg: Duel Prescaler/Counter2/Half Adder7 ==
  A : Inport
  "B " : Inport  Port=2
  AND : Logic  IconShape=distinctive  AllPortsSameDT=off  OutDataTypeStr=boolean
  XOR : Logic  Operator=XOR  IconShape=distinctive  AllPortsSameDT=off  OutDataTypeStr=boolean
  Sum : Outport
  Carry : Outport  Port=2
  wires:
  A/1 -> AND/1, XOR/1
  "B "/1 -> XOR/2, AND/2
  XOR/1 -> Sum/1
  AND/1 -> Carry/1

== system Timers/Eg: Duel Prescaler/TPSA/Subsystem1 ==
  Data : Inport
  Store : Inport  Port=2
  Clock : Inport  Port=3
  Clear : Inport  Port=4
  AND : Logic  IconShape=distinctive  AllPortsSameDT=off  OutDataTypeStr=boolean
  AND1 : Logic  IconShape=distinctive  AllPortsSameDT=off  OutDataTypeStr=boolean
  D Flip-Flop : simulink_extras/Flip Flops/D Flip-Flop
  NOT : Logic  Operator=NOT  IconShape=distinctive  AllPortsSameDT=off  OutDataTypeStr=boolean
  NOT1 : Logic  Operator=NOT  IconShape=distinctive  AllPortsSameDT=off  OutDataTypeStr=boolean
  OR : Logic  Operator=OR  IconShape=distinctive  AllPortsSameDT=off  OutDataTypeStr=boolean
  Q : Outport
  !Q : Outport  Port=2
  wires:
  AND1/1 -> OR/2
  AND/1 -> OR/1
  D Flip-Flop/1 -> Q/1, AND1/2
  NOT/1 -> AND1/1
  Store/1 -> AND/2, NOT/1
  Clock/1 -> D Flip-Flop/2
  Data/1 -> AND/1
  OR/1 -> D Flip-Flop/1
  D Flip-Flop/2 -> !Q/1
  Clear/1 -> NOT1/1
  NOT1/1 -> D Flip-Flop/3

== system Timers/Eg: Duel Prescaler/TPSA/Subsystem2 ==
  Data : Inport
  Store : Inport  Port=2
  Clock : Inport  Port=3
  Clear : Inport  Port=4
  AND : Logic  IconShape=distinctive  AllPortsSameDT=off  OutDataTypeStr=boolean
  AND1 : Logic  IconShape=distinctive  AllPortsSameDT=off  OutDataTypeStr=boolean
  D Flip-Flop : simulink_extras/Flip Flops/D Flip-Flop
  NOT : Logic  Operator=NOT  IconShape=distinctive  AllPortsSameDT=off  OutDataTypeStr=boolean
  NOT1 : Logic  Operator=NOT  IconShape=distinctive  AllPortsSameDT=off  OutDataTypeStr=boolean
  OR : Logic  Operator=OR  IconShape=distinctive  AllPortsSameDT=off  OutDataTypeStr=boolean
  Q : Outport
  !Q : Outport  Port=2
  wires:
  AND1/1 -> OR/2
  AND/1 -> OR/1
  D Flip-Flop/1 -> Q/1, AND1/2
  NOT/1 -> AND1/1
  Store/1 -> AND/2, NOT/1
  Clock/1 -> D Flip-Flop/2
  Data/1 -> AND/1
  OR/1 -> D Flip-Flop/1
  D Flip-Flop/2 -> !Q/1
  Clear/1 -> NOT1/1
  NOT1/1 -> D Flip-Flop/3

== system Timers/Eg: Duel Prescaler/TPSA/Subsystem3 ==
  Data : Inport
  Store : Inport  Port=2
  Clock : Inport  Port=3
  Clear : Inport  Port=4
  AND : Logic  IconShape=distinctive  AllPortsSameDT=off  OutDataTypeStr=boolean
  AND1 : Logic  IconShape=distinctive  AllPortsSameDT=off  OutDataTypeStr=boolean
  D Flip-Flop : simulink_extras/Flip Flops/D Flip-Flop
  NOT : Logic  Operator=NOT  IconShape=distinctive  AllPortsSameDT=off  OutDataTypeStr=boolean
  NOT1 : Logic  Operator=NOT  IconShape=distinctive  AllPortsSameDT=off  OutDataTypeStr=boolean
  OR : Logic  Operator=OR  IconShape=distinctive  AllPortsSameDT=off  OutDataTypeStr=boolean
  Q : Outport
  !Q : Outport  Port=2
  wires:
  AND1/1 -> OR/2
  AND/1 -> OR/1
  D Flip-Flop/1 -> Q/1, AND1/2
  NOT/1 -> AND1/1
  Store/1 -> AND/2, NOT/1
  Clock/1 -> D Flip-Flop/2
  Data/1 -> AND/1
  OR/1 -> D Flip-Flop/1
  D Flip-Flop/2 -> !Q/1
  Clear/1 -> NOT1/1
  NOT1/1 -> D Flip-Flop/3

== system Timers/Eg: Duel Prescaler/TPSA/Subsystem4 ==
  Data : Inport
  Store : Inport  Port=2
  Clock : Inport  Port=3
  Clear : Inport  Port=4
  AND : Logic  IconShape=distinctive  AllPortsSameDT=off  OutDataTypeStr=boolean
  AND1 : Logic  IconShape=distinctive  AllPortsSameDT=off  OutDataTypeStr=boolean
  D Flip-Flop : simulink_extras/Flip Flops/D Flip-Flop
  NOT : Logic  Operator=NOT  IconShape=distinctive  AllPortsSameDT=off  OutDataTypeStr=boolean
  NOT1 : Logic  Operator=NOT  IconShape=distinctive  AllPortsSameDT=off  OutDataTypeStr=boolean
  OR : Logic  Operator=OR  IconShape=distinctive  AllPortsSameDT=off  OutDataTypeStr=boolean
  Q : Outport
  !Q : Outport  Port=2
  wires:
  AND1/1 -> OR/2
  AND/1 -> OR/1
  D Flip-Flop/1 -> Q/1, AND1/2
  NOT/1 -> AND1/1
  Store/1 -> AND/2, NOT/1
  Clock/1 -> D Flip-Flop/2
  Data/1 -> AND/1
  OR/1 -> D Flip-Flop/1
  D Flip-Flop/2 -> !Q/1
  Clear/1 -> NOT1/1
  NOT1/1 -> D Flip-Flop/3

== system Timers/Eg: Duel Prescaler/TPSA/Subsystem5 ==
  Data : Inport
  Store : Inport  Port=2
  Clock : Inport  Port=3
  Clear : Inport  Port=4
  AND : Logic  IconShape=distinctive  AllPortsSameDT=off  OutDataTypeStr=boolean
  AND1 : Logic  IconShape=distinctive  AllPortsSameDT=off  OutDataTypeStr=boolean
  D Flip-Flop : simulink_extras/Flip Flops/D Flip-Flop
  NOT : Logic  Operator=NOT  IconShape=distinctive  AllPortsSameDT=off  OutDataTypeStr=boolean
  NOT1 : Logic  Operator=NOT  IconShape=distinctive  AllPortsSameDT=off  OutDataTypeStr=boolean
  OR : Logic  Operator=OR  IconShape=distinctive  AllPortsSameDT=off  OutDataTypeStr=boolean
  Q : Outport
  !Q : Outport  Port=2
  wires:
  AND1/1 -> OR/2
  AND/1 -> OR/1
  D Flip-Flop/1 -> Q/1, AND1/2
  NOT/1 -> AND1/1
  Store/1 -> AND/2, NOT/1
  Clock/1 -> D Flip-Flop/2
  Data/1 -> AND/1
  OR/1 -> D Flip-Flop/1
  D Flip-Flop/2 -> !Q/1
  Clear/1 -> NOT1/1
  NOT1/1 -> D Flip-Flop/3

== system Timers/Eg: Duel Prescaler/TPSA/Subsystem6 ==
  Data : Inport
  Store : Inport  Port=2
  Clock : Inport  Port=3
  Clear : Inport  Port=4
  AND : Logic  IconShape=distinctive  AllPortsSameDT=off  OutDataTypeStr=boolean
  AND1 : Logic  IconShape=distinctive  AllPortsSameDT=off  OutDataTypeStr=boolean
  D Flip-Flop : simulink_extras/Flip Flops/D Flip-Flop
  NOT : Logic  Operator=NOT  IconShape=distinctive  AllPortsSameDT=off  OutDataTypeStr=boolean
  NOT1 : Logic  Operator=NOT  IconShape=distinctive  AllPortsSameDT=off  OutDataTypeStr=boolean
  OR : Logic  Operator=OR  IconShape=distinctive  AllPortsSameDT=off  OutDataTypeStr=boolean
  Q : Outport
  !Q : Outport  Port=2
  wires:
  AND1/1 -> OR/2
  AND/1 -> OR/1
  D Flip-Flop/1 -> Q/1, AND1/2
  NOT/1 -> AND1/1
  Store/1 -> AND/2, NOT/1
  Clock/1 -> D Flip-Flop/2
  Data/1 -> AND/1
  OR/1 -> D Flip-Flop/1
  D Flip-Flop/2 -> !Q/1
  Clear/1 -> NOT1/1
  NOT1/1 -> D Flip-Flop/3

== system Timers/Eg: Duel Prescaler/TPSA/Subsystem7 ==
  Data : Inport
  Store : Inport  Port=2
  Clock : Inport  Port=3
  Clear : Inport  Port=4
  AND : Logic  IconShape=distinctive  AllPortsSameDT=off  OutDataTypeStr=boolean
  AND1 : Logic  IconShape=distinctive  AllPortsSameDT=off  OutDataTypeStr=boolean
  D Flip-Flop : simulink_extras/Flip Flops/D Flip-Flop
  NOT : Logic  Operator=NOT  IconShape=distinctive  AllPortsSameDT=off  OutDataTypeStr=boolean
  NOT1 : Logic  Operator=NOT  IconShape=distinctive  AllPortsSameDT=off  OutDataTypeStr=boolean
  OR : Logic  Operator=OR  IconShape=distinctive  AllPortsSameDT=off  OutDataTypeStr=boolean
  Q : Outport
  !Q : Outport  Port=2
  wires:
  AND1/1 -> OR/2
  AND/1 -> OR/1
  D Flip-Flop/1 -> Q/1, AND1/2
  NOT/1 -> AND1/1
  Store/1 -> AND/2, NOT/1
  Clock/1 -> D Flip-Flop/2
  Data/1 -> AND/1
  OR/1 -> D Flip-Flop/1
  D Flip-Flop/2 -> !Q/1
  Clear/1 -> NOT1/1
  NOT1/1 -> D Flip-Flop/3

== system Timers/Eg: Duel Prescaler/TPSA/Subsystem8 ==
  Data : Inport
  Store : Inport  Port=2
  Clock : Inport  Port=3
  Clear : Inport  Port=4
  AND : Logic  IconShape=distinctive  AllPortsSameDT=off  OutDataTypeStr=boolean
  AND1 : Logic  IconShape=distinctive  AllPortsSameDT=off  OutDataTypeStr=boolean
  D Flip-Flop : simulink_extras/Flip Flops/D Flip-Flop
  NOT : Logic  Operator=NOT  IconShape=distinctive  AllPortsSameDT=off  OutDataTypeStr=boolean
  NOT1 : Logic  Operator=NOT  IconShape=distinctive  AllPortsSameDT=off  OutDataTypeStr=boolean
  OR : Logic  Operator=OR  IconShape=distinctive  AllPortsSameDT=off  OutDataTypeStr=boolean
  Q : Outport
  !Q : Outport  Port=2
  wires:
  AND1/1 -> OR/2
  AND/1 -> OR/1
  D Flip-Flop/1 -> Q/1, AND1/2
  NOT/1 -> AND1/1
  Store/1 -> AND/2, NOT/1
  Clock/1 -> D Flip-Flop/2
  Data/1 -> AND/1
  OR/1 -> D Flip-Flop/1
  D Flip-Flop/2 -> !Q/1
  Clear/1 -> NOT1/1
  NOT1/1 -> D Flip-Flop/3

== system Timers/Eg: Duel Prescaler/TPSB/Subsystem1 ==
  Data : Inport
  Store : Inport  Port=2
  Clock : Inport  Port=3
  Clear : Inport  Port=4
  AND : Logic  IconShape=distinctive  AllPortsSameDT=off  OutDataTypeStr=boolean
  AND1 : Logic  IconShape=distinctive  AllPortsSameDT=off  OutDataTypeStr=boolean
  D Flip-Flop : simulink_extras/Flip Flops/D Flip-Flop
  NOT : Logic  Operator=NOT  IconShape=distinctive  AllPortsSameDT=off  OutDataTypeStr=boolean
  NOT1 : Logic  Operator=NOT  IconShape=distinctive  AllPortsSameDT=off  OutDataTypeStr=boolean
  OR : Logic  Operator=OR  IconShape=distinctive  AllPortsSameDT=off  OutDataTypeStr=boolean
  Q : Outport
  !Q : Outport  Port=2
  wires:
  AND1/1 -> OR/2
  AND/1 -> OR/1
  D Flip-Flop/1 -> Q/1, AND1/2
  NOT/1 -> AND1/1
  Store/1 -> AND/2, NOT/1
  Clock/1 -> D Flip-Flop/2
  Data/1 -> AND/1
  OR/1 -> D Flip-Flop/1
  D Flip-Flop/2 -> !Q/1
  Clear/1 -> NOT1/1
  NOT1/1 -> D Flip-Flop/3

== system Timers/Eg: Duel Prescaler/TPSB/Subsystem2 ==
  Data : Inport
  Store : Inport  Port=2
  Clock : Inport  Port=3
  Clear : Inport  Port=4
  AND : Logic  IconShape=distinctive  AllPortsSameDT=off  OutDataTypeStr=boolean
  AND1 : Logic  IconShape=distinctive  AllPortsSameDT=off  OutDataTypeStr=boolean
  D Flip-Flop : simulink_extras/Flip Flops/D Flip-Flop
  NOT : Logic  Operator=NOT  IconShape=distinctive  AllPortsSameDT=off  OutDataTypeStr=boolean
  NOT1 : Logic  Operator=NOT  IconShape=distinctive  AllPortsSameDT=off  OutDataTypeStr=boolean
  OR : Logic  Operator=OR  IconShape=distinctive  AllPortsSameDT=off  OutDataTypeStr=boolean
  Q : Outport
  !Q : Outport  Port=2
  wires:
  AND1/1 -> OR/2
  AND/1 -> OR/1
  D Flip-Flop/1 -> Q/1, AND1/2
  NOT/1 -> AND1/1
  Store/1 -> AND/2, NOT/1
  Clock/1 -> D Flip-Flop/2
  Data/1 -> AND/1
  OR/1 -> D Flip-Flop/1
  D Flip-Flop/2 -> !Q/1
  Clear/1 -> NOT1/1
  NOT1/1 -> D Flip-Flop/3

== system Timers/Eg: Duel Prescaler/TPSB/Subsystem3 ==
  Data : Inport
  Store : Inport  Port=2
  Clock : Inport  Port=3
  Clear : Inport  Port=4
  AND : Logic  IconShape=distinctive  AllPortsSameDT=off  OutDataTypeStr=boolean
  AND1 : Logic  IconShape=distinctive  AllPortsSameDT=off  OutDataTypeStr=boolean
  D Flip-Flop : simulink_extras/Flip Flops/D Flip-Flop
  NOT : Logic  Operator=NOT  IconShape=distinctive  AllPortsSameDT=off  OutDataTypeStr=boolean
  NOT1 : Logic  Operator=NOT  IconShape=distinctive  AllPortsSameDT=off  OutDataTypeStr=boolean
  OR : Logic  Operator=OR  IconShape=distinctive  AllPortsSameDT=off  OutDataTypeStr=boolean
  Q : Outport
  !Q : Outport  Port=2
  wires:
  AND1/1 -> OR/2
  AND/1 -> OR/1
  D Flip-Flop/1 -> Q/1, AND1/2
  NOT/1 -> AND1/1
  Store/1 -> AND/2, NOT/1
  Clock/1 -> D Flip-Flop/2
  Data/1 -> AND/1
  OR/1 -> D Flip-Flop/1
  D Flip-Flop/2 -> !Q/1
  Clear/1 -> NOT1/1
  NOT1/1 -> D Flip-Flop/3

== system Timers/Eg: Duel Prescaler/TPSB/Subsystem4 ==
  Data : Inport
  Store : Inport  Port=2
  Clock : Inport  Port=3
  Clear : Inport  Port=4
  AND : Logic  IconShape=distinctive  AllPortsSameDT=off  OutDataTypeStr=boolean
  AND1 : Logic  IconShape=distinctive  AllPortsSameDT=off  OutDataTypeStr=boolean
  D Flip-Flop : simulink_extras/Flip Flops/D Flip-Flop
  NOT : Logic  Operator=NOT  IconShape=distinctive  AllPortsSameDT=off  OutDataTypeStr=boolean
  NOT1 : Logic  Operator=NOT  IconShape=distinctive  AllPortsSameDT=off  OutDataTypeStr=boolean
  OR : Logic  Operator=OR  IconShape=distinctive  AllPortsSameDT=off  OutDataTypeStr=boolean
  Q : Outport
  !Q : Outport  Port=2
  wires:
  AND1/1 -> OR/2
  AND/1 -> OR/1
  D Flip-Flop/1 -> Q/1, AND1/2
  NOT/1 -> AND1/1
  Store/1 -> AND/2, NOT/1
  Clock/1 -> D Flip-Flop/2
  Data/1 -> AND/1
  OR/1 -> D Flip-Flop/1
  D Flip-Flop/2 -> !Q/1
  Clear/1 -> NOT1/1
  NOT1/1 -> D Flip-Flop/3

== system Timers/Eg: Duel Prescaler/TPSB/Subsystem5 ==
  Data : Inport
  Store : Inport  Port=2
  Clock : Inport  Port=3
  Clear : Inport  Port=4
  AND : Logic  IconShape=distinctive  AllPortsSameDT=off  OutDataTypeStr=boolean
  AND1 : Logic  IconShape=distinctive  AllPortsSameDT=off  OutDataTypeStr=boolean
  D Flip-Flop : simulink_extras/Flip Flops/D Flip-Flop
  NOT : Logic  Operator=NOT  IconShape=distinctive  AllPortsSameDT=off  OutDataTypeStr=boolean
  NOT1 : Logic  Operator=NOT  IconShape=distinctive  AllPortsSameDT=off  OutDataTypeStr=boolean
  OR : Logic  Operator=OR  IconShape=distinctive  AllPortsSameDT=off  OutDataTypeStr=boolean
  Q : Outport
  !Q : Outport  Port=2
  wires:
  AND1/1 -> OR/2
  AND/1 -> OR/1
  D Flip-Flop/1 -> Q/1, AND1/2
  NOT/1 -> AND1/1
  Store/1 -> AND/2, NOT/1
  Clock/1 -> D Flip-Flop/2
  Data/1 -> AND/1
  OR/1 -> D Flip-Flop/1
  D Flip-Flop/2 -> !Q/1
  Clear/1 -> NOT1/1
  NOT1/1 -> D Flip-Flop/3
